simulink model "dspadpcm"  (Simulink 5.0)
settings: Solver=ode5  SolverMode=SingleTasking  StartTime=0.0  StopTime=.1999  FixedStep=1/64000  MaxStep=1/64000  RelTol=1e-3  AbsTol=1e-6
libraries: dspsigops x3, dspwvfmcdlib x1, dsparch3 x1, simulink3 x1
settings Model: Creator=don  LastModifiedBy=mkhan  ExtModeTrigMode=oneshot  ExtModeArmWhenConnect=off  SaveTime=off  SaveOutput=off  LimitDataPoints=off  SignalLoggingName=logsOut  IntegerOverflowMsg=none  BlockReductionOpt=off  BooleanDataType=off  ZeroCrossControl=UseLocalSettings  TargetHWChar=2  TargetHWWordLengths=8,16,32,32  RTWMathFcnLibMatFile=iso_c_tmw.mat  RTWOptions="-aEnforceIntegerDowncast=1 -aFoldNonRolledExpr=1 -aInlineInvariantSignals=1 -aInlineParameters=0 -aLocalBlockOutputs=1 -aRollThreshold=2 -aRTWVerbose=1 -aForceParamTrailComments=0 -aGenerateComments=1 -aIgnoreCustomStorageClasses=1 -aIncHierarchyInIds=0 -aMaxRTWIdLen=31 -aShowEliminatedStatements=0 -aReadOnly=0 -aTargetFcnLib=\"iso_c_tmw.mat\" -aIncDataTypeInIds=0 -aPrefixModelToSubsysFcnNames=1 -aInlinedPrmAccess=\"Literals\" -aGenerateFullHeader=1 -aIsPILTarget=0 -aGenerateReport=0 -aLogVarNameModifier=\"rt_\" -aExtMode=0 -aExtModeStaticAlloc=0 -aExtModeTesting=0 -aExtModeStaticAllocSize=1000000 -aExtModeTransport=0"

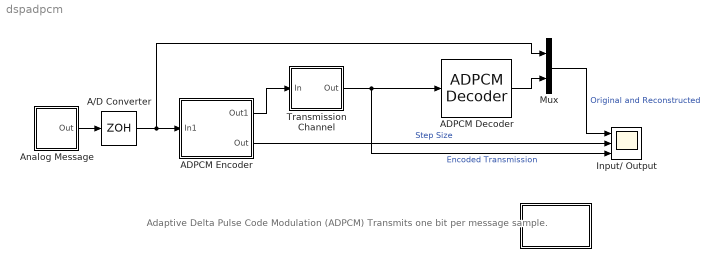
== system dspadpcm ==
  note: Adaptive Delta
      | Pulse Code Modulation (ADPCM)
      |
      | Transmits one bit per message sample.
  " " : Subsystem
      mask Type: ADPCM Demo Info
      mask Display: disp('Info')
  A/D Converter : ZeroOrderHold  SampleTime=1/8000
  ADPCM Decoder : dspwvfmcdlib/ADPCM Decoder  StepAttn=.5  StepGain=2  StepMax=0.5  StepMin=0.01  StepInit=0.1  AdpcmIntTau=0.99
  ADPCM Encoder : Subsystem  AncestorBlock=dspwvfmcdlib/ADPCM Encoder  mask(ADPCM Encoder){EncStepAttn=.5, EncStepGain=2, EncStepMax=0.5, EncStepMin=0.01, EncStepInit=0.1, EncIntTau=0.99}
      mask prompts: EncStepAttn "Step-size attenuation"; EncStepGain "Step-size gain"; EncStepMax "Maximum step size"; EncStepMin "Minimum step size"; EncStepInit "Initial step size"; EncIntTau "Integrator time constant"
      mask Display: disp('ADPCM\nEncoder')
  Analog Message : Subsystem
  Input/ Output : Scope  NumInputPorts=3
      settings: TimeRange=0.02  YMin=-1.25~-0.75~-1.2  YMax=1.25~0.75~1.2  DataFormat=Array
  Mux : Mux  Inputs=2
  Transmission Channel : Subsystem
  wires:
  Mux/1 -> Input/ Output/1  "Original and Reconstructed"
  Transmission Channel/1(Out) -> ADPCM Decoder/1, Input/ Output/3  "Encoded Transmission"
  A/D Converter/1 -> Mux/1, ADPCM Encoder/1(In1)
  Analog Message/1(Out) -> A/D Converter/1
  ADPCM Decoder/1 -> Mux/2
  ADPCM Encoder/1(Out1) -> Transmission Channel/1(In)
  ADPCM Encoder/2(Out) -> Input/ Output/2  "Step Size"

== system dspadpcm/  ==
  note: Adaptive Delta Modulation (ADM)
      |
      | Adaptive Delta Modulation (ADM) is a modification of Delta Modulation (DM).
      | DM is a differential waveform quantization (or coding) technique.
      | A DM encoder uses the error between the original signal to be
      | coded and the coded signal itself to create a differentially-quantized data stream.
      | This data stream (usually the computer error signal) is a lower-bit-rate signal that can be
      | decoded by a matched decoder on the receiver side in order to achieve data
      | compression and hence low data transmission rates.
      |
      | ADM employs a two-level (i.e. one bit) encoders, and may be performed
      | at many different sampling/data rates. ADM has a variable step-size.
      | Each "1" bit means "increase the amplitude" by the step size as compared
      | to previous decoded signal sample, while a  "0" bit means
      | "decrease the amplitude" by the step-size. Thus when slope overload occurs the step
      | size becomes progressively larger, thereby allowing the re-constructed signal to catch
      | up with the original signal more rapidly. Conversely, when the input signal slope
      | changes slowly, the step-size is decreased.

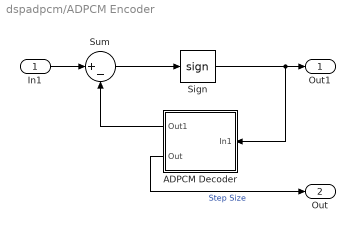
== system dspadpcm/ADPCM Encoder ==
  In1 : Inport
  ADPCM Decoder : Subsystem  Orientation=left  AncestorBlock=dspwvfmcdlib/ADPCM Decoder  mask(ADPCM Decoder){StepAttn=EncStepAttn, StepGain=EncStepGain, StepMax=EncStepMax, StepMin=EncStepMin, StepInit=EncStepInit, AdpcmIntTau=EncIntTau}
      mask prompts: StepAttn "Step-size attenuation"; StepGain "Step-size gain"; StepMax "Maximum step size"; StepMin "Minimum step size"; StepInit "Initial step size"; AdpcmIntTau "Integrator time constant"
      mask Display: disp('ADPCM\nDecoder')
  Sign : Signum
  Sum : Sum  Inputs=|+-  SaturateOnIntegerOverflow=on  InputSameDT=on
  Out1 : Outport
  Out : Outport  Port=2
  wires:
  ADPCM Decoder/1(Out1) -> Sum/2
  Sum/1 -> Sign/1
  Sign/1 -> ADPCM Decoder/1(In1), Out1/1
  In1/1 -> Sum/1
  ADPCM Decoder/2(Out) -> Out/1  "Step Size"

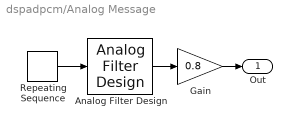
== system dspadpcm/Analog Message ==
  Analog Filter Design : dsparch3/Analog Filter Design  method=Butterworth  filttype=Lowpass  N=5  Wlo=2*pi*400  Whi=80  Rp=2  Rs=40
  Gain : Gain  Gain=0.8  SaturateOnIntegerOverflow=on
  Repeating Sequence : simulink3/Sources/Repeating Sequence  rep_seq_t=[0 .005 .005 .015 .015 .02]  rep_seq_y=[1 1 -1 -1 1 1]
  Out : Outport  InitialOutput=0
  wires:
  Analog Filter Design/1 -> Gain/1
  Repeating Sequence/1 -> Analog Filter Design/1
  Gain/1 -> Out/1

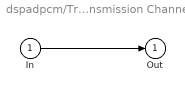
== system dspadpcm/Transmission Channel ==
  In : Inport
  Out : Outport  InitialOutput=0
  wires:
  In/1 -> Out/1

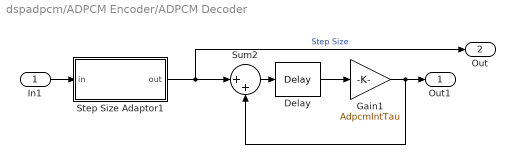
== system dspadpcm/ADPCM Encoder/ADPCM Decoder ==
  In1 : Inport
  Delay : dspsigops/Delay  dly_unit=Samples  delay=1  ic_detail=on  dif_ic_for_ch=off  dif_ic_for_dly=off  ic=0  reset_popup=None
  Gain1 : Gain  Gain=AdpcmIntTau  SaturateOnIntegerOverflow=on
  Step Size Adaptor1 : Subsystem  mask(Step-size adaptation){Dec=StepAttn, Inc=StepGain, MaxStep=StepMax, MinStep=StepMin, InitStep=StepInit}
      mask prompts: Dec "Step-size attenuation factor:"; Inc "Step-size gain factor:"; MaxStep "Maximum step size:"; MinStep "Minimum step size:"; InitStep "Initial step size:"
      mask help: Step-size logic
      mask Display: disp('Step Size\nAdaptation')
  Sum2 : Sum  Inputs=|++  SaturateOnIntegerOverflow=on  InputSameDT=on
  Out1 : Outport
  Out : Outport  Port=2
  wires:
  In1/1 -> Step Size Adaptor1/1(in)
  Delay/1 -> Gain1/1
  Sum2/1 -> Delay/1
  Step Size Adaptor1/1(out) -> Sum2/1, Out/1  "Step Size"
  Gain1/1 -> Out1/1, Sum2/2

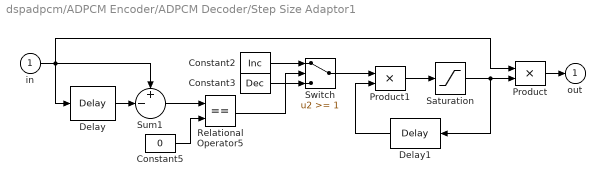
== system dspadpcm/ADPCM Encoder/ADPCM Decoder/Step Size Adaptor1 ==
  in : Inport
  Constant2 : Constant  Value=Inc
  Constant3 : Constant  Value=Dec
  Constant5 : Constant  Value=0
  Delay : dspsigops/Delay  dly_unit=Samples  delay=1  ic_detail=on  dif_ic_for_ch=off  dif_ic_for_dly=off  ic=0  reset_popup=None
  Delay1 : dspsigops/Delay  Orientation=left  dly_unit=Samples  delay=1  ic_detail=on  dif_ic_for_ch=off  dif_ic_for_dly=off  ic=0  reset_popup=None
  Product : Product  SaturateOnIntegerOverflow=on  RndMeth=Zero  InputSameDT=on
  Product1 : Product  SaturateOnIntegerOverflow=on  RndMeth=Zero  InputSameDT=on
  Relational Operator5 : RelationalOperator  Operator===  InputSameDT=on
  Saturation : Saturate  UpperLimit=MaxStep  LowerLimit=MinStep
  Sum1 : Sum  Inputs=+-|  SaturateOnIntegerOverflow=on  InputSameDT=on
  Switch : Switch  Threshold=1  SaturateOnIntegerOverflow=on  InputSameDT=on
  out : Outport  InitialOutput=0
  wires:
  Constant5/1 -> Relational Operator5/2
  Delay/1 -> Sum1/2
  in/1 -> Product/1, Sum1/1, Delay/1
  Delay1/1 -> Product1/2
  Switch/1 -> Product1/1
  Product1/1 -> Saturation/1
  Sum1/1 -> Relational Operator5/1
  Constant3/1 -> Switch/3
  Constant2/1 -> Switch/1
  Relational Operator5/1 -> Switch/2
  Product/1 -> out/1
  Saturation/1 -> Product/2, Delay1/1
